simulink subsystem "LowLevelController1"  (R2023a)
settings: Solver=VariableStepAuto  StartTime=0.0  StopTime=10.0  RelTol=1e-3
settings Model: Creator=stude  LastModifiedBy=stude

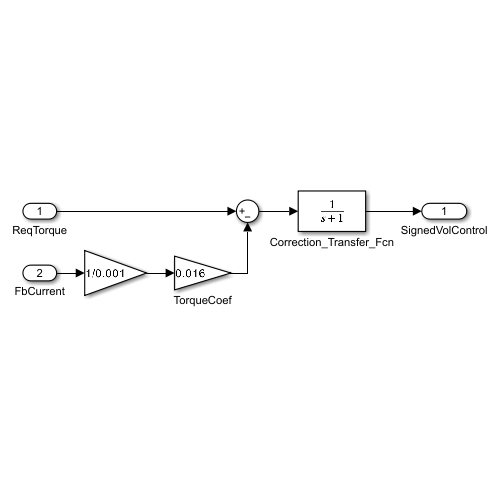
[thumbnail: Simulink's stored preview of the top-level diagram]
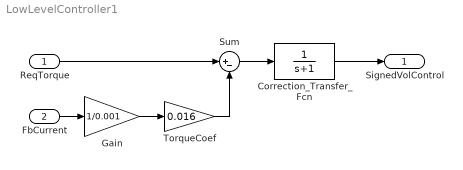
== system LowLevelController1 ==
  ReqTorque : Inport
  FbCurrent : Inport  Port=2
  Correction_Transfer_Fcn : TransferFcn  Denominator=[1 1]
  Gain : Gain  Gain=1/0.001
  Sum : Sum  Inputs=|+-
  TorqueCoef : Gain  Gain=0.016
  SignedVolControl : Outport
  wires:
  Correction_Transfer_Fcn/1 -> SignedVolControl/1
  ReqTorque/1 -> Sum/1
  FbCurrent/1 -> Gain/1
  TorqueCoef/1 -> Sum/2
  Sum/1 -> Correction_Transfer_Fcn/1
  Gain/1 -> TorqueCoef/1
